simulink model "FSKDemodulator"  (R2024a)
settings: Solver=VariableStepAuto  StartTime=0.0  StopTime=10.0  RelTol=1e-3
settings Model: Creator=prath  LastModifiedBy=prath

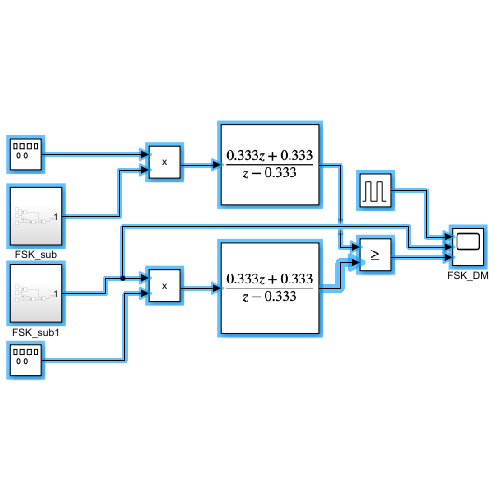
[thumbnail: Simulink's stored preview of the top-level diagram]
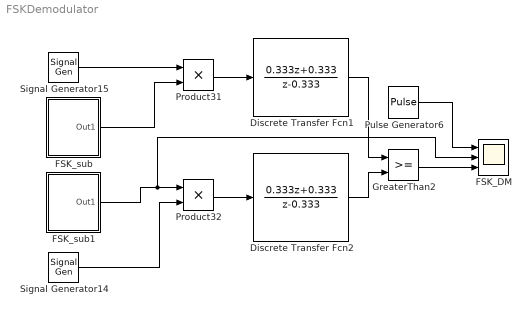
== system FSKDemodulator ==
  Discrete Transfer Fcn1 : DiscreteTransferFcn  Numerator=[0.333 0.333]  Denominator=[1 -0.333]
  Discrete Transfer Fcn2 : DiscreteTransferFcn  Numerator=[0.333 0.333]  Denominator=[1 -0.333]
  FSK_DM : Scope  NumInputPorts=3
  FSK_sub : Subsystem
  FSK_sub1 : Subsystem
  GreaterThan2 : RelationalOperator  OutDataTypeStr=boolean  RndMeth=Simplest  InputSameDT=off
  Product31 : Product
  Product32 : Product
  Pulse Generator6 : DiscretePulseGenerator  PulseType=Time based  PulseWidth=50
  Signal Generator14 : SignalGenerator  Frequency=5
  Signal Generator15 : SignalGenerator  Frequency=20
  wires:
  Signal Generator14/1 -> Product32/2
  Discrete Transfer Fcn1/1 -> GreaterThan2/1
  Product32/1 -> Discrete Transfer Fcn2/1
  GreaterThan2/1 -> FSK_DM/3
  Pulse Generator6/1 -> FSK_DM/1
  FSK_sub1/1(Out1) -> FSK_DM/2, Product32/1
  FSK_sub/1(Out1) -> Product31/2
  Product31/1 -> Discrete Transfer Fcn1/1
  Signal Generator15/1 -> Product31/1
  Discrete Transfer Fcn2/1 -> GreaterThan2/2

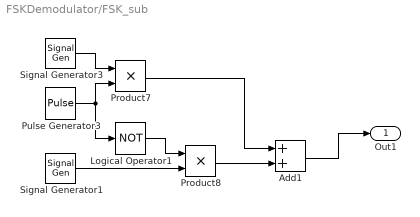
== system FSKDemodulator/FSK_sub ==
  Add1 : Sum
  Logical Operator1 : Logic  Operator=NOT  IconShape=distinctive  AllPortsSameDT=off  OutDataTypeStr=boolean
  Product7 : Product
  Product8 : Product
  Pulse Generator3 : DiscretePulseGenerator  PulseType=Time based  PulseWidth=50
  Signal Generator1 : SignalGenerator  Frequency=5
  Signal Generator3 : SignalGenerator  Frequency=20
  Out1 : Outport
  wires:
  Signal Generator1/1 -> Product8/2
  Pulse Generator3/1 -> Logical Operator1/1, Product7/2
  Product7/1 -> Add1/1
  Logical Operator1/1 -> Product8/1
  Signal Generator3/1 -> Product7/1
  Product8/1 -> Add1/2
  Add1/1 -> Out1/1

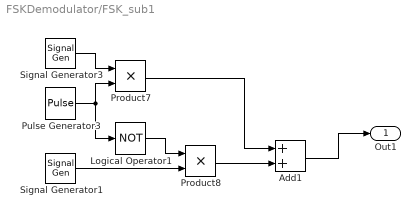
== system FSKDemodulator/FSK_sub1 ==
  Add1 : Sum
  Logical Operator1 : Logic  Operator=NOT  IconShape=distinctive  AllPortsSameDT=off  OutDataTypeStr=boolean
  Product7 : Product
  Product8 : Product
  Pulse Generator3 : DiscretePulseGenerator  PulseType=Time based  PulseWidth=50
  Signal Generator1 : SignalGenerator  Frequency=5
  Signal Generator3 : SignalGenerator  Frequency=20
  Out1 : Outport
  wires:
  Signal Generator1/1 -> Product8/2
  Pulse Generator3/1 -> Logical Operator1/1, Product7/2
  Product7/1 -> Add1/1
  Logical Operator1/1 -> Product8/1
  Signal Generator3/1 -> Product7/1
  Product8/1 -> Add1/2
  Add1/1 -> Out1/1
